simulink model "BlockDiagram_WhiteBox"  (R2025b)
settings: Solver=VariableStepAuto  StartTime=0.0  StopTime=10.0  RelTol=1e-3
settings Model: Creator=gruby  LastModifiedBy=gruby

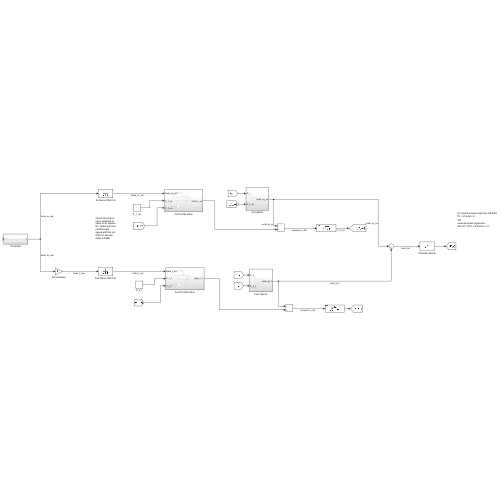
[thumbnail: Simulink's stored preview of the top-level diagram]
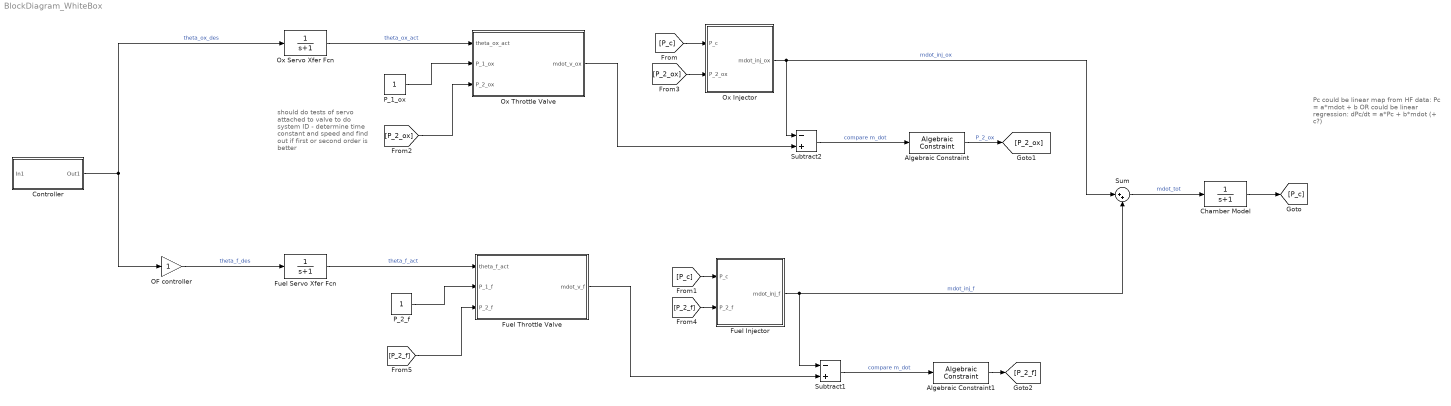
== system BlockDiagram_WhiteBox ==
  note: should do tests of servo attached to valve to do system ID - determine time constant and speed and find out if first or second order is better
  note: Pc could be linear map from HF data:
      | Pc = a*mdot + b
      | OR
      | could be linear regression:
      | dPc/dt = a*Pc + b*mdot (+ c?)
  Algebraic Constraint : AlgebraicConstraint
  Algebraic Constraint1 : AlgebraicConstraint
  Chamber Model : TransferFcn  Denominator=[1 1]
  Controller : Subsystem
  Fuel Injector : Subsystem
  Fuel Servo Xfer Fcn : TransferFcn  Denominator=[1 1]
  Fuel Throttle Valve : Subsystem
  OF controller : Gain
  Ox Injector : Subsystem
  Ox Servo Xfer Fcn : TransferFcn  Denominator=[1 1]
  Ox Throttle Valve : Subsystem
  P_1_ox : Constant
  P_2_f : Constant
  Subtract1 : Sum  Inputs=-+
  Subtract2 : Sum  Inputs=-+
  Sum : Sum  Inputs=|++
  wires:
  Subtract2/1 -> Algebraic Constraint/1  "compare m_dot"
  Ox Throttle Valve/1(mdot_v_ox) -> Subtract2/2
  Ox Injector/1(mdot_inj_ox) -> Sum/1, Subtract2/1  "mdot_inj_ox"
  Subtract1/1 -> Algebraic Constraint1/1  "compare m_dot"
  Fuel Injector/1(mdot_inj_f) -> Sum/2, Subtract1/1  "mdot_inj_f"
  Fuel Throttle Valve/1(mdot_v_f) -> Subtract1/2
  Sum/1 -> Chamber Model/1  "mdot_tot"
  Chamber Model/1 -> [P_c]
  [P_c] -> Ox Injector/1(P_c)
  [P_c] -> Fuel Injector/1(P_c)
  Algebraic Constraint/1 -> [P_2_ox]  "P_2_ox"
  [P_2_ox] -> Ox Throttle Valve/3(P_2_ox)
  [P_2_ox] -> Ox Injector/2(P_2_ox)
  Algebraic Constraint1/1 -> [P_2_f]
  [P_2_f] -> Fuel Injector/2(P_2_f)
  [P_2_f] -> Fuel Throttle Valve/3(P_2_f)
  P_1_ox/1 -> Ox Throttle Valve/2(P_1_ox)
  P_2_f/1 -> Fuel Throttle Valve/2(P_1_f)
  Ox Servo Xfer Fcn/1 -> Ox Throttle Valve/1(theta_ox_act)  "theta_ox_act"
  Fuel Servo Xfer Fcn/1 -> Fuel Throttle Valve/1(theta_f_act)  "theta_f_act"
  Controller/1(Out1) -> OF controller/1, Ox Servo Xfer Fcn/1  "theta_ox_des"
  OF controller/1 -> Fuel Servo Xfer Fcn/1  "theta_f_des"

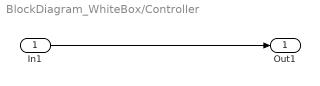
== system BlockDiagram_WhiteBox/Controller ==
  In1 : Inport
  Out1 : Outport
  wires:
  In1/1 -> Out1/1

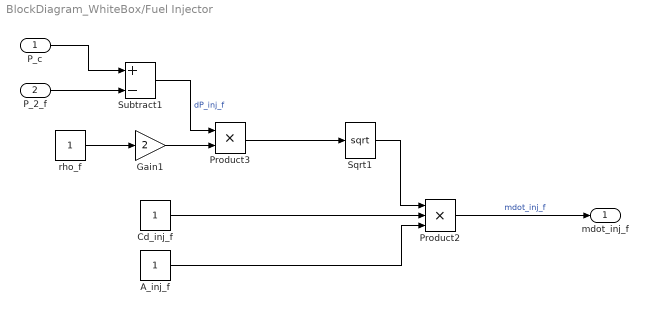
== system BlockDiagram_WhiteBox/Fuel Injector ==
  P_c : Inport
  P_2_f : Inport  Port=2
  A_inj_f : Constant
  Cd_inj_f : Constant
  Gain1 : Gain  Gain=2
  Product2 : Product  Inputs=3
  Product3 : Product
  Sqrt1 : Sqrt
  Subtract1 : Sum  Inputs=+-
  rho_f : Constant
  mdot_inj_f : Outport
  wires:
  Subtract1/1 -> Product3/1  "dP_inj_f"
  Cd_inj_f/1 -> Product2/2
  rho_f/1 -> Gain1/1
  P_2_f/1 -> Subtract1/2
  Product3/1 -> Sqrt1/1
  Sqrt1/1 -> Product2/1
  Gain1/1 -> Product3/2
  A_inj_f/1 -> Product2/3
  P_c/1 -> Subtract1/1
  Product2/1 -> mdot_inj_f/1  "mdot_inj_f"

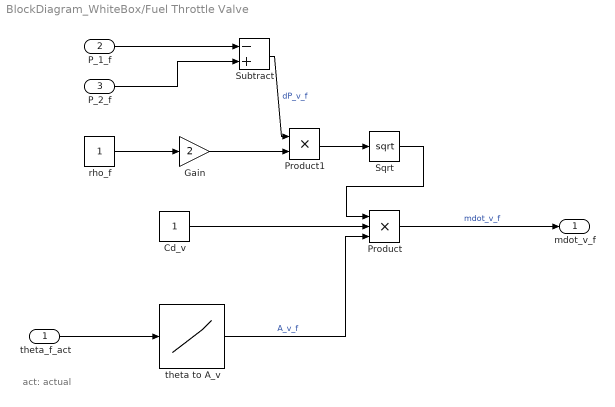
== system BlockDiagram_WhiteBox/Fuel Throttle Valve ==
  note: act: actual
  theta_f_act : Inport
  P_1_f : Inport  Port=2
  P_2_f : Inport  Port=3
  Cd_v : Constant
  Gain : Gain  Gain=2
  Product : Product  Inputs=3
  Product1 : Product
  Sqrt : Sqrt
  Subtract : Sum  Inputs=-+
  rho_f : Constant
  theta to A_v : Lookup_n-D  NumberOfTableDimensions=1  BreakpointsForDimension1=[-5:5]  Table=tanh([-5:5])  InternalRulePriority=Speed  RndMeth=Simplest
  mdot_v_f : Outport
  wires:
  Subtract/1 -> Product1/1  "dP_v_f"
  Sqrt/1 -> Product/1
  rho_f/1 -> Gain/1
  Product/1 -> mdot_v_f/1  "mdot_v_f"
  Gain/1 -> Product1/2
  theta to A_v/1 -> Product/3  "A_v_f"
  Cd_v/1 -> Product/2
  Product1/1 -> Sqrt/1
  theta_f_act/1 -> theta to A_v/1
  P_2_f/1 -> Subtract/2
  P_1_f/1 -> Subtract/1

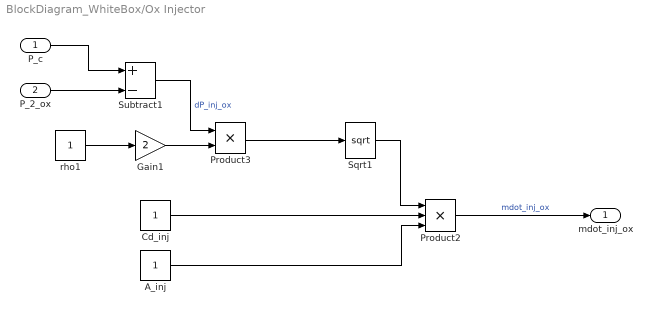
== system BlockDiagram_WhiteBox/Ox Injector ==
  P_c : Inport
  P_2_ox : Inport  Port=2
  A_inj : Constant
  Cd_inj : Constant
  Gain1 : Gain  Gain=2
  Product2 : Product  Inputs=3
  Product3 : Product
  Sqrt1 : Sqrt
  Subtract1 : Sum  Inputs=+-
  rho1 : Constant
  mdot_inj_ox : Outport
  wires:
  Subtract1/1 -> Product3/1  "dP_inj_ox"
  Cd_inj/1 -> Product2/2
  rho1/1 -> Gain1/1
  P_2_ox/1 -> Subtract1/2
  Product3/1 -> Sqrt1/1
  Sqrt1/1 -> Product2/1
  Gain1/1 -> Product3/2
  A_inj/1 -> Product2/3
  P_c/1 -> Subtract1/1
  Product2/1 -> mdot_inj_ox/1  "mdot_inj_ox"

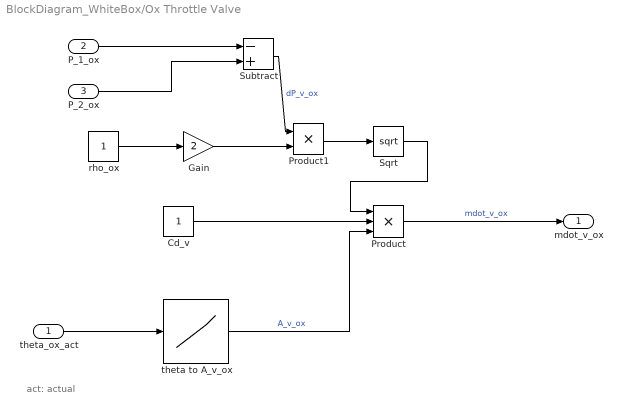
== system BlockDiagram_WhiteBox/Ox Throttle Valve ==
  note: act: actual
  theta_ox_act : Inport
  P_1_ox : Inport  Port=2
  P_2_ox : Inport  Port=3
  Cd_v : Constant
  Gain : Gain  Gain=2
  Product : Product  Inputs=3
  Product1 : Product
  Sqrt : Sqrt
  Subtract : Sum  Inputs=-+
  rho_ox : Constant
  theta to A_v_ox : Lookup_n-D  NumberOfTableDimensions=1  BreakpointsForDimension1=[-5:5]  Table=tanh([-5:5])  InternalRulePriority=Speed  RndMeth=Simplest
  mdot_v_ox : Outport
  wires:
  Subtract/1 -> Product1/1  "dP_v_ox"
  Sqrt/1 -> Product/1
  rho_ox/1 -> Gain/1
  Product/1 -> mdot_v_ox/1  "mdot_v_ox"
  Gain/1 -> Product1/2
  theta to A_v_ox/1 -> Product/3  "A_v_ox"
  Cd_v/1 -> Product/2
  Product1/1 -> Sqrt/1
  theta_ox_act/1 -> theta to A_v_ox/1
  P_1_ox/1 -> Subtract/1
  P_2_ox/1 -> Subtract/2
